simulink model ""  (R2025a)
settings: Solver=VariableStepAuto  StartTime=0.0  StopTime=2  RelTol=1e-3
values from neighbouring files (symbols this model uses):
  Ts = T(T.classCode == 0, :)    [sweep_exp3_KB_Td_stg1_clean.m]    (also in sweep_exp3_KB_Td_stg2_clean.m)
undefined symbols (not defined in the file or in its folder): b_eq, Bc, I_eq, k_eq, Kc, r_h, r_p, r_s, vM0, vS0, xM0, xS0
settings Model: Creator=ekaitz  LastModifiedBy=ekaitz

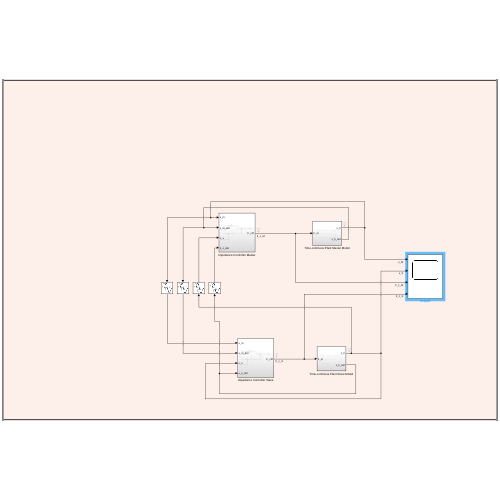
[thumbnail: Simulink's stored preview of the top-level diagram]
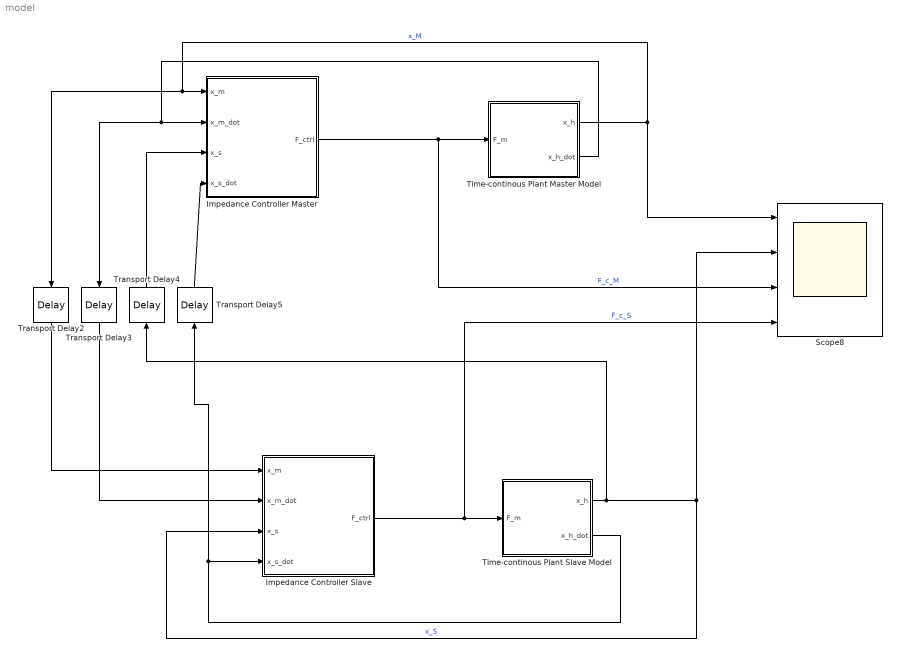
== system model ==
  Impedance Controller Master : Subsystem
  Impedance Controller Slave : Subsystem
  Scope8 : Scope  NumInputPorts=4
      settings: ActiveDisplayYMinimum=-0.0018144396114250845  ActiveDisplayYMaximum=0.0057571599568250094  DataLoggingVariableName=ScopeData7
  Time-continous Plant Master Model : Subsystem
  Time-continous Plant Slave Model : Subsystem
  Transport Delay{2..5} (4 alike) : TransportDelay  DelayTime=Ts
  wires:
  Transport Delay5/1 -> Impedance Controller Master/4(x_s_dot)
  Time-continous Plant Slave Model/1(x_h) -> Scope8/2, Impedance Controller Slave/3(x_s), Transport Delay4/1  "x_S"
  Impedance Controller Slave/1(F_ctrl) -> Time-continous Plant Slave Model/1(F_m), Scope8/4  "F_c_S"
  Impedance Controller Master/1(F_ctrl) -> Scope8/3, Time-continous Plant Master Model/1(F_m)  "F_c_M"
  Transport Delay3/1 -> Impedance Controller Slave/2(x_m_dot)
  Transport Delay4/1 -> Impedance Controller Master/3(x_s)
  Time-continous Plant Master Model/1(x_h) -> Transport Delay2/1, Impedance Controller Master/1(x_m), Scope8/1  "x_M"
  Transport Delay2/1 -> Impedance Controller Slave/1(x_m)
  Time-continous Plant Slave Model/2(x_h_dot) -> Impedance Controller Slave/4(x_s_dot), Transport Delay5/1
  Time-continous Plant Master Model/2(x_h_dot) -> Transport Delay3/1, Impedance Controller Master/2(x_m_dot)

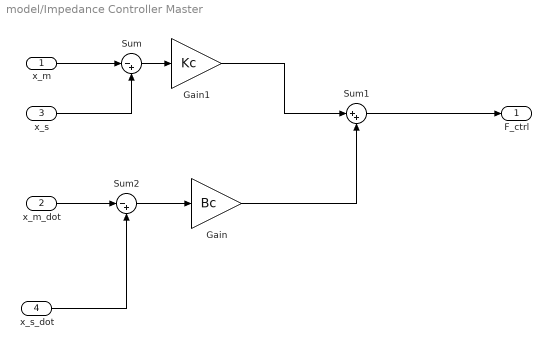
== system model/Impedance Controller Master ==
  x_m : Inport
  x_m_dot : Inport  Port=2
  x_s : Inport  Port=3
  x_s_dot : Inport  Port=4
  Gain : Gain  Gain=Bc
  Gain1 : Gain  Gain=Kc
  Sum : Sum  Inputs=|-+
  Sum1 : Sum  Inputs=|++
  Sum2 : Sum  Inputs=|-+
  F_ctrl : Outport
  wires:
  x_m/1 -> Sum/1
  Sum/1 -> Gain1/1
  Gain1/1 -> Sum1/1
  Gain/1 -> Sum1/2
  x_s/1 -> Sum/2
  x_m_dot/1 -> Sum2/1
  x_s_dot/1 -> Sum2/2
  Sum2/1 -> Gain/1
  Sum1/1 -> F_ctrl/1

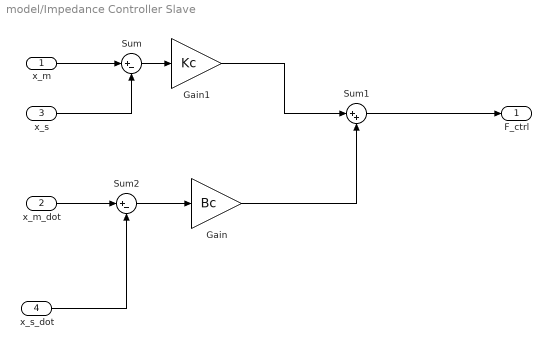
== system model/Impedance Controller Slave ==
  x_m : Inport
  x_m_dot : Inport  Port=2
  x_s : Inport  Port=3
  x_s_dot : Inport  Port=4
  Gain : Gain  Gain=Bc
  Gain1 : Gain  Gain=Kc
  Sum : Sum  Inputs=|+-
  Sum1 : Sum  Inputs=|++
  Sum2 : Sum  Inputs=|+-
  F_ctrl : Outport
  wires:
  x_m/1 -> Sum/1
  Sum/1 -> Gain1/1
  Gain1/1 -> Sum1/1
  Gain/1 -> Sum1/2
  x_s/1 -> Sum/2
  x_m_dot/1 -> Sum2/1
  x_s_dot/1 -> Sum2/2
  Sum2/1 -> Gain/1
  Sum1/1 -> F_ctrl/1

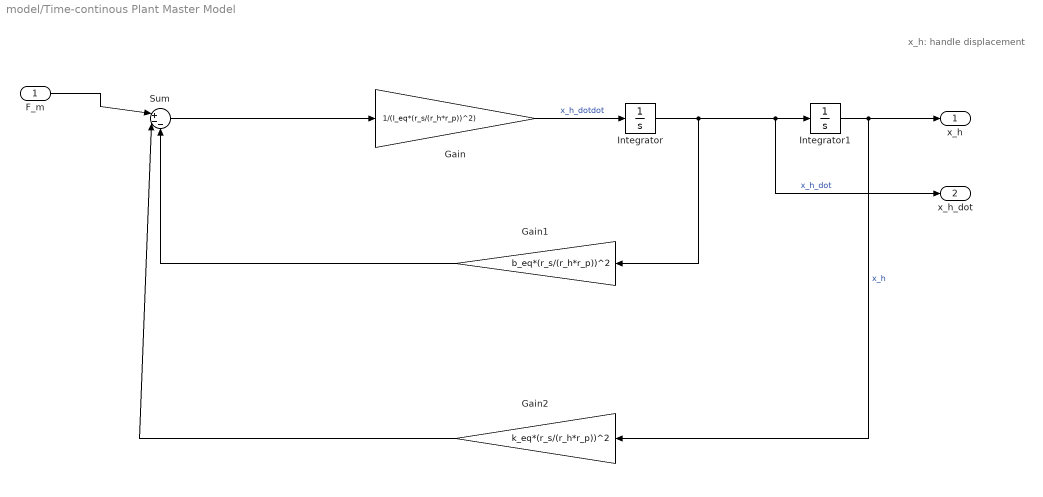
== system model/Time-continous Plant Master Model ==
  note: x_h: handle displacement
  F_m : Inport
  Gain : Gain  Gain=1/(I_eq*(r_s/(r_h*r_p))^2)
  Gain1 : Gain  Gain=b_eq*(r_s/(r_h*r_p))^2
  Gain2 : Gain  Gain=k_eq*(r_s/(r_h*r_p))^2
  Integrator : Integrator  InitialCondition=vM0
  Integrator1 : Integrator  InitialCondition=xM0
  Sum : Sum  Inputs=|+--
  x_h : Outport
  x_h_dot : Outport  Port=2
  wires:
  Gain2/1 -> Sum/2
  Gain/1 -> Integrator/1  "x_h_dotdot"
  F_m/1 -> Sum/1
  Integrator1/1 -> x_h/1, Gain2/1  "x_h"
  Gain1/1 -> Sum/3
  Sum/1 -> Gain/1
  Integrator/1 -> Gain1/1, x_h_dot/1, Integrator1/1  "x_h_dot"

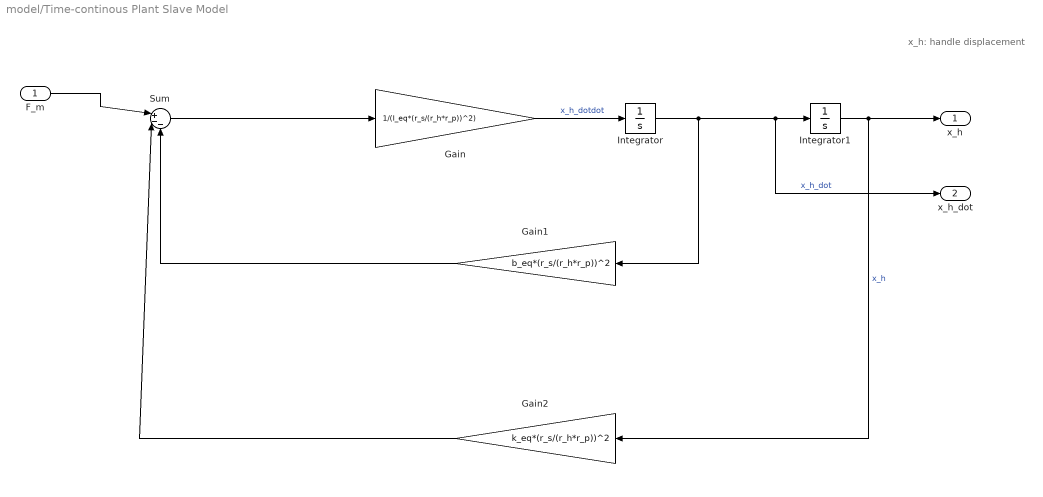
== system model/Time-continous Plant Slave Model ==
  note: x_h: handle displacement
  F_m : Inport
  Gain : Gain  Gain=1/(I_eq*(r_s/(r_h*r_p))^2)
  Gain1 : Gain  Gain=b_eq*(r_s/(r_h*r_p))^2
  Gain2 : Gain  Gain=k_eq*(r_s/(r_h*r_p))^2
  Integrator : Integrator  InitialCondition=vS0
  Integrator1 : Integrator  InitialCondition=xS0
  Sum : Sum  Inputs=|+--
  x_h : Outport
  x_h_dot : Outport  Port=2
  wires:
  Gain2/1 -> Sum/2
  Gain/1 -> Integrator/1  "x_h_dotdot"
  F_m/1 -> Sum/1
  Integrator1/1 -> x_h/1, Gain2/1  "x_h"
  Gain1/1 -> Sum/3
  Sum/1 -> Gain/1
  Integrator/1 -> Gain1/1, x_h_dot/1, Integrator1/1  "x_h_dot"
